simulink model "exercise02_simulation_model_template"  (R2025b)
settings: Solver=ode45  StartTime=0.0  StopTime=10  FixedStep=1e-5  MaxStep=1e-3  RelTol=1e-4  EnableMultiTasking=on
PreLoadFcn:
  | exercise02_simulation_parameters
values from neighbouring files (symbols this model uses):
  g = 9.81    [exercise03_solution_compute_LQR_outer_loop_controller.m]
undefined symbols (not defined in the file or in its folder): cmd_2_newtons_conversion_linear_coefficient, cmd_2_newtons_conversion_quadratic_coefficient, cmd_max, cmd_min, DiscIntNeverNeededParam, K_lqr, measurement_noise, nrotor_initial_conditions, nrotor_vehicle, pid_x, pid_y, pid_z, reference, sample_time, sigbuilder_block
libraries: simulink x3
(part 2 of 2)

== matlab function exercise02_simulation_model_template/N-rotor vehicle model/Full equations of motions implemented in one shot/The full equations of motion implemented with one function ==
  data: g input; full_state_dot output; m input; J input; J_inv input; layout input; thrusts input; full_state input; body_rates output; body_accel output
function [full_state_dot,body_rates,body_accel] = fcn_eom(g,m,J,J_inv,layout,thrusts,full_state)
%
% ----------------------------------------------------------------------- %
% DESCRIPTION:
% This function implements the full equation of motion in one function to
% simplify the exposition.
%
%
% INPUT ARGUMENTS:
% m
% > This is the mass of the vehicle, in units of kilograms
%
% g
% > This is the acceleration due to gravity (typically 9.81), in units of
%   meters per second squared
%
% J
% > This is the moment of inertia matrix of the vehicle (it should be a
%   3-by3 matrix), the units of each element is kilogram meters squared
%
% J_inv
% > This is the inverse of the momement of inertia matrix, it is not
%   compute in this script to reduce the simulation run time slightly
%
% layout
% > This is a matrix that specifies the layout via the following format:
% nrotor_vehicle_layout = [...
%       x_1  ,  x_2  ,  ...  ,  x_{N-1}  ,  x_{N}  ;...
%       y_1  ,  y_2  ,  ...  ,  y_{N-1}  ,  y_{N}  ;...
%       c_1  ,  c_2  ,  ...  ,  c_{N-1}  ,  c_{N}   ...
%   ];
% where:
%   > x_i   is the x coordinate of propeller "i" relative to the CoG
%   > y_i   is the y coordinate of propeller "i" relative to the CoG
%   > c_i   is the thurst to torque coefficient of the propeller, with the
%           sign used to indicate the propeller's direction of rotation,
%           +ve indicates clock-wise propeller rotation.
%
% thrusts
% > This is a colulmn vector with length equal to the number of propellers
%   on the N-rotor vehicle, and each element represents the thrust force in
%   Newtons being produced by the respective propeller
%
% full_state
% > This is a vector of length 12 and is order as:
%   full_state[1:3]     the x,y,z posiiton of the body frame origin
%                       expressed in inertial frame coordinates, in units
%                       of [meters].
%
%   full_state[4:6]     the x,y,z linear velocity of the body frame origin
%                       expressed in inertial frame coordinates, in units
%                       of [meters per second].
%
%   full_state[7:9]     the roll, pitch, and yaw intrinsic Euler angles
%                       respectively, in units of [radians].
%
%   full_state[10:12]   the angular velocity of the roll, pitch, and yaw
%                       intrinsic Euler angles respectively, in units of
%                       [radians per second].
%
%
% RETURN ARGUMENTS:
% full_state_dot
% > This is a vector of length 12 and is ordered as:
%   full_state_dot[1:3]
%      - This is position dot and is taken directly as full_state[4:6]
%
%   full_state_dot[4:6]
%      - This is the position double dot and is computed using the equation
%        of motion for transaltion, it has units of [meters per second
%        squared]
%
%   full_state_dot[7:9]
%      - This is the angular velocity of the intrinsic Euler angles and is
%        taken directly as full_state[10:12]
%
%   full_state_dot[10:12]
%      - This is the angular accelerations of the intrinsic Euler angles
%        and is computed using the equation of motion for Euler angle
%        rotations, it has units of [radians per second squared]
%
% body_rates
% > This is a vector of length 3, each element represents the angular
%   velocity of the body frame as measured about the body frame's
%   coordinate axes, ordered as:
%   body_rates = [ w_x ; w_y ; w_z ];
%   In other words, this is exactly what is measured by a typical
%   strap-down Inertial Measurement Unit (IMU) that is attached to the body
%   of most all flying vehicles. It is computed directly from the "psi_dot"
%   by that is extracted from the "full_state" by applying the
%   transformation matrix "T". It has units of [radians per second];
%
% body_accel
% > This is a vector of length 3, each element represents the linear
%   accelerations of the body frame as measured along the body frame's
%   coordinate axes, i.e., this is exctly what is measured by a typical
%   strap-down Inertial Measurement Unit (IMU). It is computed directly
%   from the "pos_double_dot" by applying the rotation matrix from inertial
%   to body frame. It has units of [meters per second squared].
%
% ----------------------------------------------------------------------- %


% Extract the components of the full state
%pos      =  full_state(1:3);
pos_dot  =  full_state(4:6);
psi      =  full_state(7:9);
psi_dot  =  full_state(10:12);


% Extract each Euler angles
roll   =  psi(1);  % Roll  (gamma is the symbol used in the script)
pitch  =  psi(2);  % Pitch (beta  is the symbol used in the script)
yaw    =  psi(3);  % Yaw   (alpha is the symbol used in the script)


% Extract each Euler anglular rates
roll_dot   =  psi_dot(1);  % Roll  angular velocity
pitch_dot  =  psi_dot(2);  % Pitch angular velocity
%yaw_dot    =  psi_dot(3); % Yaw   angular velocity, not needed


% Compute the rotation matrix from body frame to inertial frame:
R_B2I = [...
            cos(yaw)*cos(pitch)  ,...
                cos(yaw)*sin(pitch)*sin(roll)-sin(yaw)*cos(roll)  ,...
                cos(yaw)*sin(pitch)*cos(roll)+sin(yaw)*sin(roll)   ...
            ;...
            sin(yaw)*cos(pitch)  ,...
                sin(yaw)*sin(pitch)*sin(roll)+cos(yaw)*cos(roll)  ,...
                sin(yaw)*sin(pitch)*cos(roll)-cos(yaw)*sin(roll)   ...
            ;...
            -sin(pitch)  ,...
                cos(pitch)*sin(roll)  ,...
                cos(pitch)*cos(roll)   ...
    ];


% Compute the T matrix:
T = [...
        1  ,  0          ,  -sin(pitch)            ;...
        0  ,  cos(roll)  ,   sin(roll)*cos(pitch)  ;...
        0  , -sin(roll)  ,   cos(roll)*cos(pitch)   ...
    ];


% Compute the T inverse matrix:
T_inv = [...
        1  ,  sin(roll)*tan(pitch)  ,   cos(roll)*tan(pitch)  ;...
        0  ,  cos(roll)             ,  -sin(roll)             ;...
        0  ,  sin(roll)*sec(pitch)  ,   cos(roll)*sec(pitch)   ...
    ];


% Compute the time derivative of the T matrix:
T_dot = [...
        0  ,   0                   ,  -pitch_dot*cos(pitch)                                          ;...
        0  ,  -roll_dot*sin(roll)  ,   roll_dot*cos(roll)*cos(pitch)-pitch_dot*sin(roll)*sin(pitch)  ;...
        0  ,  -roll_dot*cos(roll)  ,  -roll_dot*sin(roll)*cos(pitch)-pitch_dot*cos(roll)*sin(pitch)   ...
    ];


% Implement the equation of motion for translation
pos_double_dot = (1/m) .* ( R_B2I * [0;0;sum(thrusts(:))] ) + [0;0;-g];


% Compute the body rates from the Euler angluar rates
w = T * psi_dot;


% Implement the equation of motion for body frame rotations
w_dot = J_inv * ( [layout(2,:);-layout(1,:);layout(3,:)] * thrusts - cross( w , J*w ) );


% Implement the equation of motion for Euler angle rotations
psi_double_dot = T_inv * ( w_dot - T_dot * psi_dot );


% Put together the "full_state_dot" return variable
full_state_dot = [...
        pos_dot ;...
        pos_double_dot ;...
        psi_dot ;...
        psi_double_dot ...
    ];


% Put together the "body_rates" return variable
body_rates = w;


% Finally compute the accelerations in the body frame
% > by "simply" rotating the inertial frame linear accelerations, i.e.,
%   "pos_double_dot", from the inertial frame into the body frame
% > do you need to account for the fact that the body frame accelerations
%   are measured in a rotating frame?
body_accel = transpose(R_B2I) * psi_double_dot;


end

== matlab function exercise02_simulation_model_template/Controller/outer control loop/compute the per-propeller thrust desired ==
  data: thrusts_for_equilibrium input; additional_thrust_desired input; thrusts_per_motor output
function thrusts_per_motor = compute_per_motor_thrust( thrusts_for_equilibrium , additional_thrust_desired )
% ----------------------------------------------------------------------- %
% DESCRIPTION:
% This function computes the desired thrust per propeller that provides the
% total thrust and body frame (x,y,z) torques requested for an N-rotor
% vehicle with a particular layout
%
%
% INPUT ARGUMENTS:
% thrusts_for_equilibrium
% > This is a colulmn vector with length equal to the number of propellers
%   on the N-rotor vehicle, and each element represents the thrust force in
%   Newtons that will maintain the N-rotor vehicle at the hover equilibrium
%
% additional_thrust_desired [Newtons]
% > This is the total additional thrust force desired
%
%
% RETURN ARGUMENTS:
% thrusts_per_motor
% > This is a colulmn vector with length equal to the number of propellers
%   on the N-rotor vehicle, and each element represents the thrust force in
%   Newtons that is desired from the respective propeller
%
%
% ----------------------------------------------------------------------- %

% Compute any residual thrust that results from the "thrusts_for_torque"
total_equilibrium_thrust = sum( thrusts_for_equilibrium(:) );

% Compute the desired thrust per propeller:
thrusts_per_motor = thrusts_for_equilibrium * ...
    ( (additional_thrust_desired+total_equilibrium_thrust)/total_equilibrium_thrust );

== matlab function exercise02_simulation_model_template/Controller/outer control loop/MATLAB Function ==
  data: current_yaw input; xy_error_in_inertial_frame input; xy_error_in_body_frame output
function xy_error_in_body_frame = rotate_xy_intertial_to_body( current_yaw , xy_error_in_inertial_frame )
% ----------------------------------------------------------------------- %
% DESCRIPTION:
% This function rotates an (x,y) coordainte and (x_dot,y_dot) velocity
% vector from the interial frame into (approximately) the body frame. The
% approximate is because the rotation into the body frame is only based on
% the current yaw of the vehicle and assumes that roll and pitch are zero.
%
%
% INPUT ARGUMENTS:
% current_yaw
% > The intrinsic Euler yaw angle, in radians
%
% xy_error_in_inertial_frame [m;m;m/s;m/s]
% > The measurement of (x,y) position and velocities in the inertial frame
%
%
% RETURN ARGUMENTS:
% xy_error_in_body_frame
% > The measurement of (x,y) position and velocities rotated into the body
%   frame
%
%
% ----------------------------------------------------------------------- %


% Extract the inertial position and velocities
x_I      =  xy_error_in_inertial_frame(1);
y_I      =  xy_error_in_inertial_frame(2);
xdot_I   =  xy_error_in_inertial_frame(3);
ydot_I   =  xy_error_in_inertial_frame(4);


% Initialise the return variable "xy_error_in_body_frame" to zeros
% > This can be required so that Simulink knows the expected size
xy_error_in_body_frame = zeros(4,1);


% Rotate the inertial POSITIONS into the body frame
% > For computing x in the body frame
xy_error_in_body_frame(1,1) =  +x_I;
% > For computing y in the body frame
xy_error_in_body_frame(2,1) =  +y_I;


% Rotate the inertial VELOCITIES into the body frame
% > For computing xdot in the body frame
xy_error_in_body_frame(3,1) =  +xdot_I;
% > For computing ydot in the body frame
xy_error_in_body_frame(4,1) =  +ydot_I;
